simulink model "tarefa12"  (R2022b)
settings: Solver=VariableStepAuto  StartTime=0.0  StopTime=30.0  RelTol=1e-3
values from neighbouring files (symbols this model uses):
  Cd = [0 1.092]    [lab12.m]
  d = -0.15    [lab12.m]
  F = [0.001 -0.382; 0.35 0.739]    [lab12.m]
  H = [0.35;0.239]    [lab12.m]
  K = place(F,H,[0.834+0.172i, 0.834-0.172i])    [lab12.m]
  L = L_T'    [lab12.m]
  R = 1.25    [lab12.m]
  T0 = 0.377    [lab12.m]
  td = 15    [lab12.m]
  X0_OBS = [0 0]    [lab12.m]
  X0_SIS = [-0.15 0.15]    [lab12.m]
settings Model: Creator=hugo_  LastModifiedBy=hugo_

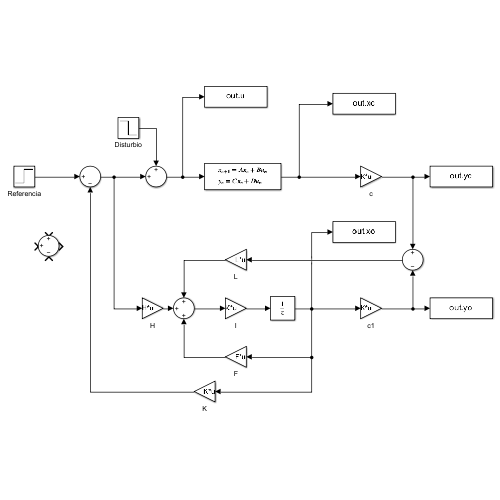
[thumbnail: Simulink's stored preview of the top-level diagram]
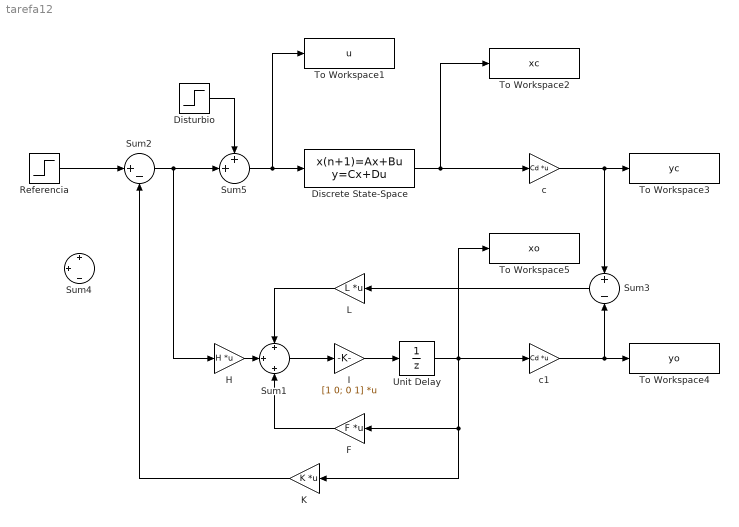
== system tarefa12 ==
  Discrete State-Space : DiscreteStateSpace  A=F  B=H  C=[1 0; 0 1]  D=[0;0]  InitialCondition=X0_SIS  SampleTime=T0
  Disturbio : Step  Time=td  After=d  SampleTime=0
  F : Gain  Gain=F  Multiplication=Matrix(K*u)
  H : Gain  Gain=H  Multiplication=Matrix(K*u)
  I : Gain  Gain=[1 0; 0 1]  Multiplication=Matrix(K*u)
  K : Gain  Gain=K  Multiplication=Matrix(K*u)
  L : Gain  Gain=L  Multiplication=Matrix(K*u)
  Referencia : Step  Time=0  After=R  SampleTime=0
  Sum1 : Sum  Inputs=+|+|+
  Sum2 : Sum  Inputs=|+-
  Sum3 : Sum  Inputs=+|-
  Sum4 : Sum  Inputs=+|+|-
  Sum5 : Sum  Inputs=++|
  To Workspace1 : ToWorkspace  VariableName=u  SaveFormat=Timeseries  SampleTime=-1
  To Workspace2 : ToWorkspace  VariableName=xc  SaveFormat=Timeseries  SampleTime=-1
  To Workspace3 : ToWorkspace  VariableName=yc  SaveFormat=Timeseries  SampleTime=-1
  To Workspace4 : ToWorkspace  VariableName=yo  SaveFormat=Timeseries  SampleTime=-1
  To Workspace5 : ToWorkspace  VariableName=xo  SaveFormat=Timeseries  SampleTime=-1
  Unit Delay : UnitDelay  InitialCondition=X0_OBS  SampleTime=T0  HasFrameUpgradeWarning=on
  c : Gain  Gain=Cd  Multiplication=Matrix(K*u)
  c1 : Gain  Gain=Cd  Multiplication=Matrix(K*u)
  wires:
  L/1 -> Sum1/1
  Unit Delay/1 -> To Workspace5/1, c1/1, K/1, F/1
  Sum3/1 -> L/1
  c1/1 -> To Workspace4/1, Sum3/2
  I/1 -> Unit Delay/1
  Sum1/1 -> I/1
  Discrete State-Space/1 -> To Workspace2/1, c/1
  H/1 -> Sum1/2
  Sum2/1 -> Sum5/2, H/1
  c/1 -> Sum3/1, To Workspace3/1
  F/1 -> Sum1/3
  Referencia/1 -> Sum2/1
  K/1 -> Sum2/2
  Disturbio/1 -> Sum5/1
  Sum5/1 -> To Workspace1/1, Discrete State-Space/1
